simulink model "P2_SIL_Model_Diag"  (R2016a)
settings: Solver=ode2  StartTime=0.0  StopTime=Cycle_End  RelTol=1e-3
undefined symbols (not defined in the file): air, APP1_OOR, APP2_OOR, APP_Conversion_IN, APP_Mismatch, bms_inletair_temp, bms_maxchargecurrent, bms_maxdischargecurrent, BMS_Notfallkuehlung, BPP_Flt, cal, clt, ClutchEngag, CrankRequest, dcdc, eng, Engine, EngOverTemp, ENGTRQ_MSMCH_Degraded_CP, ENGTRQ_MSMCH_ErrCritical_CP, ENGTRQ_MSMCH_LimpHome_CP, EngTrqMismatch, env, ess, ESS, ESSOverTemp, fd, FFD, g, gb, Grade, IMG, KeyPos_Flt, KeyPosition, lib_APP_Conversion_IN, lib_ESS_plant_V1_2, lib_OBC_Manager, LossCAN, max_vehicle_rad_air_flow, MCUOverTemp, mot, MotDirMismatch, MotOverTemp, MotTrqMismatch, mph2kph, mph2ms, NeutralGear, obc, OBC_Manager, ParkGear, PRNDL_Flt, ReverseGear, RFD, rho, ShiftLeverPosition, sigbuilder_block, Speed, t_amb, time, tloop ... (+2)
libraries: simulink x104, EC2_libraries x12, Diagnostic x11, lib_CANerror_Detect x3, Utility x1
(part 3 of 11)

== system P2_SIL_Model_Diag/Actuators/CAN/HV_CAN/MCU ==
  In1 : Inport
  Bus Creator : BusCreator  Inputs=4
  Bus Selector : BusSelector  OutputSignals=MCU_CAN,Controls.Torque_Command,Controls.Inverter_Enable,Controls.ClutchEngage
  Out1 : Outport
  wires:
  In1/1 -> Bus Selector/1
  Bus Selector/1 -> Bus Creator/1  "<MCU_CAN>"
  Bus Selector/2 -> Bus Creator/2  "<Torque_Command>"
  Bus Creator/1 -> Out1/1
  Bus Selector/3 -> Bus Creator/3  "<Inverter_Enable>"
  Bus Selector/4 -> Bus Creator/4  "<ClutchEngage>"

== system P2_SIL_Model_Diag/Actuators/CAN/HV_CAN/OBC ==
  In1 : Inport
  Bus Selector : BusSelector  OutputSignals=OBC_CAN
  Out1 : Outport
  wires:
  In1/1 -> Bus Selector/1
  Bus Selector/1 -> Out1/1  "<OBC_CAN>"

== system P2_SIL_Model_Diag/Actuators/CAN/VEH_CAN/BCM ==
  In1 : Inport
  Bus Creator : BusCreator  Inputs=2
  Bus Selector : BusSelector  OutputSignals=Controls.powerMode,Controls.SysPwrMd
  Memory : Memory
  Out1 : Outport
  wires:
  In1/1 -> Bus Selector/1
  Bus Selector/1 -> Bus Creator/1  "<powerMode>"
  Bus Selector/2 -> Memory/1  "<SysPwrMd>"
  Bus Creator/1 -> Out1/1
  Memory/1 -> Bus Creator/2  "SysPwrMd"

== system P2_SIL_Model_Diag/Actuators/CAN/VEH_CAN/EBCM ==
  In1 : Inport
  Out1 : Outport
  wires:
  In1/1 -> Out1/1

== system P2_SIL_Model_Diag/Actuators/CAN/VEH_CAN/ICCM ==
  In1 : Inport
  Out1 : Outport
  wires:
  In1/1 -> Out1/1

== system P2_SIL_Model_Diag/Actuators/CAN/VEH_CAN/TCM ==
  In1 : Inport
  Bus Creator : BusCreator  Inputs=2
  Bus Selector : BusSelector  OutputSignals=Controls.VehSpdAvgDrvn_kph,Controls.AccPos_Perc
  Out1 : Outport
  wires:
  In1/1 -> Bus Selector/1
  Bus Selector/1 -> Bus Creator/1  "<VehSpdAvgDrvn_kph>"
  Bus Selector/2 -> Bus Creator/2  "<AccPos_Perc>"
  Bus Creator/1 -> Out1/1

== system P2_SIL_Model_Diag/Camaro Plant Model/Differential/Torque calculation/Blending (state dependent) ==
  Input : Inport
  Control (state) : Inport  Port=2
  Linear spline : Fcn  Expr=(u<xl)*yl + (xl<=u)*(u<xc)*((yc-yl)*(u-xl)/(xc-xl)+yl) + (xc<=u)*(u<xr)*((yc-yr)*(u-xr)/(xc-xr)+yr) + (xr<=u)*yr
  Product2 : Product  SaturateOnIntegerOverflow=on  InputSameDT=on  OutDataTypeStr=Inherit: Same as first input
  Output : Outport
  wires:
  Input/1 -> Product2/1
  Linear spline/1 -> Product2/2
  Product2/1 -> Output/1
  Control (state)/1 -> Linear spline/1

== system P2_SIL_Model_Diag/Camaro Plant Model/Differential/Torque calculation/Look-Up Table (2-D) ==
  Rows : Inport
  Cols : Inport  Port=2
  Look-Up Table (2-D) : Lookup2D  RowIndex=x  ColumnIndex=y  Table=t  SaturateOnIntegerOverflow=on  InputSameDT=on
  Out1 : Outport
  wires:
  Rows/1 -> Look-Up Table (2-D)/1
  Cols/1 -> Look-Up Table (2-D)/2
  Look-Up Table (2-D)/1 -> Out1/1

== system P2_SIL_Model_Diag/Camaro Plant Model/ESS/ESS/ESSThermal ==
  note: TempDeltaCdeg
  Resistance : Inport
  Current : Inport  Port=2
  BatteryMass : Constant  Value=ess.plant.init.bat_mass
  Constant : Constant  Value=0.01
  Divide : Product  Inputs=*/
  LowerLimit : Subsystem  mask{Lolimit=t_amb}
      mask prompts: Lolimit "Lower Limit:"
  LowerLimit1 : Subsystem  mask{Lolimit=70000}
      mask prompts: Lolimit "Lower Limit:"
  Memory : Memory  X0=t_amb
  Multiply : Product  Inputs=3
  Product : Product  RndMeth=Zero
  SpecificHeatCapBattery : Constant  Value=ess.plant.init.specific_heat
  Sum : Sum  Inputs=|++
  Sum1 : Sum  Inputs=-++  SaturateOnIntegerOverflow=on  InputSameDT=on  OutDataTypeStr=Inherit: Same as first input
  Sum2 : Sum  SaturateOnIntegerOverflow=on  InputSameDT=on  OutDataTypeStr=Inherit: Same as first input
  Switch4 : Switch  Threshold=1
  To Workspace3 : ToWorkspace  VariableName=ess_temp_hist  SampleTime=-1
      settings: Decimation=WORKSPACE_DECIMATION
  To_WHr1 : Gain  Gain=tloop  SaturateOnIntegerOverflow=on  OutDataTypeStr=Inherit: Same as input  ParamDataTypeStr=Inherit: Same as input
  To_WHr2 : Gain  Gain=5  SaturateOnIntegerOverflow=on  OutDataTypeStr=Inherit: Same as input  ParamDataTypeStr=Inherit: Same as input
  Temp[degC] : Outport
  wires:
  Sum2/1 -> Sum1/1
  Constant/1 -> Sum2/2  "NaturalCooling"
  [ESS_WEGPmp] -> Sum2/1
  To_WHr1/1 -> Divide/1  "d(Wh)"
  Current/1 -> Multiply/1, Multiply/2
  Resistance/1 -> Multiply/3
  Sum1/1 -> To_WHr1/1
  LowerLimit/1(Out) -> To Workspace3/1, Memory/1, Temp[degC]/1
  Memory/1 -> Sum/2
  Sum/1 -> LowerLimit/1(In)
  Divide/1 -> Sum/1
  BatteryMass/1 -> Product/1  "kg"
  SpecificHeatCapBattery/1 -> Product/2  "J/kg*K"
  Product/1 -> Divide/2
  Multiply/1 -> Sum1/2, To_WHr2/1  "J/s"
  Switch4/1 -> Sum1/3  "ResistiveFault"
  [ESSHighRes] -> Switch4/2, Switch4/3
  To_WHr2/1 -> LowerLimit1/1(In)
  LowerLimit1/1(Out) -> Switch4/1

== system P2_SIL_Model_Diag/Camaro Plant Model/ESS/ESS/LoadCharacteristics ==
  Current : Inport
  I*r : Product  RndMeth=Zero
  LowerLimit1 : Subsystem  mask{Lolimit=40}
      mask prompts: Lolimit "Lower Limit:"
  LowerLimit2 : Subsystem  mask{Lolimit=30}
      mask prompts: Lolimit "Lower Limit:"
  SOC Calculation : Subsystem
  Sum : Sum
  Switch1 : Switch  Threshold=1
  Switch2 : Switch
  Switch4 : Switch  Threshold=1
  To Workspace3 : ToWorkspace  VariableName=ess_voc_hist  SampleTime=-1
      settings: Decimation=WORKSPACE_DECIMATION
  To_WHr1 : Gain  Gain=10  SaturateOnIntegerOverflow=on  OutDataTypeStr=Inherit: Same as input  ParamDataTypeStr=Inherit: Same as input
  To_WHr2 : Gain  Gain=10  SaturateOnIntegerOverflow=on  OutDataTypeStr=Inherit: Same as input  ParamDataTypeStr=Inherit: Same as input
  To_WHr3 : Gain  Gain=1.01  SaturateOnIntegerOverflow=on  OutDataTypeStr=Inherit: Same as input  ParamDataTypeStr=Inherit: Same as input
  To_WHr4 : Gain  Gain=0.99  SaturateOnIntegerOverflow=on  OutDataTypeStr=Inherit: Same as input  ParamDataTypeStr=Inherit: Same as input
  resistor_charge (ohm) : Lookup  InputValues=ess.plant.init.bat_soc_idx  Table=ess.plant.init.bat_r_chg
  resistor_discharge (ohm) : Lookup  InputValues=ess.plant.init.bat_soc_idx  Table=ess.plant.init.bat_r_dis
  voc (volt) : Lookup  InputValues=ess.plant.init.bat_soc_idx  Table=ess.plant.init.bat_voc
  will use charge when >=0 : Switch
  Vterm : Outport
  Resistance : Outport  Port=2
  tag scope: SOC=global
  wires:
  To_WHr4/1 -> Switch2/1
  To_WHr3/1 -> Switch2/3
  Switch2/1 -> [Current_internal], SOC Calculation/1(Current)
  SOC Calculation/1(SOC) -> [SOC], voc (volt)/1, resistor_charge (ohm)/1, resistor_discharge (ohm)/1
  will use charge when >=0/1 -> Resistance/1, I*r/1
  I*r/1 -> Sum/2
  voc (volt)/1 -> [OCV], Sum/1, To Workspace3/1
  Sum/1 -> Vterm/1, [V_term]
  [ESSHighRes] -> Switch4/2, Switch1/2
  To_WHr2/1 -> LowerLimit1/1(In)
  resistor_charge (ohm)/1 -> Switch4/3, To_WHr2/1
  Switch4/1 -> will use charge when >=0/1  "ResistiveFault"
  Switch1/1 -> will use charge when >=0/3
  resistor_discharge (ohm)/1 -> Switch1/3, To_WHr1/1
  To_WHr1/1 -> LowerLimit2/1(In)
  LowerLimit1/1(Out) -> Switch4/1
  LowerLimit2/1(Out) -> Switch1/1
  Current/1 -> Switch2/2, To_WHr3/1, will use charge when >=0/2, I*r/2, [Current_term], To_WHr4/1

== system P2_SIL_Model_Diag/Camaro Plant Model/ESS/Inputs/CAN_fromHCU ==
  Bus Creator : BusCreator  Inputs=2
  Outputs : Outport
  wires:
  [HCU_to_HV_CAN] -> Bus Creator/1
  [HCU_to_EBCAN] -> Bus Creator/2
  Bus Creator/1 -> Outputs/1

== system P2_SIL_Model_Diag/Camaro Plant Model/ESS/Inputs/Digital_fromHCU ==
  Outputs : Outport
  wires:
  [Digital] -> Outputs/1

== system P2_SIL_Model_Diag/Camaro Plant Model/ESS/Soft BMS/BMS_06 ==
  Bus Creator8 : BusCreator  Inputs=9
  Constant2 : Constant  Value=0
  BMS_06 : Outport
  wires:
  Constant2/1 -> Bus Creator8/2  "BMS_SollVolumenStrom"
  Bus Creator8/1 -> BMS_06/1  "BMS_06"
  ? -> Bus Creator8/8
  ? -> Bus Creator8/6
  ? -> Bus Creator8/4
  ? -> Bus Creator8/3
  ? -> Bus Creator8/7
  ? -> Bus Creator8/9
  ? -> Bus Creator8/5

== system P2_SIL_Model_Diag/Camaro Plant Model/ESS/Soft BMS/BMS_07 ==
  Bus Creator8 : BusCreator  Inputs=9
  BMS_07 : Outport
  wires:
  ? -> Bus Creator8/5
  ? -> Bus Creator8/9
  ? -> Bus Creator8/7
  [BMS_Gesamtst_Spgfreiheit] -> Bus Creator8/1  "BMS_Gesamtst_Spgfreiheit"
  ? -> Bus Creator8/3
  ? -> Bus Creator8/4
  ? -> Bus Creator8/6
  ? -> Bus Creator8/8
  Bus Creator8/1 -> BMS_07/1  "BMS_07"
  ? -> Bus Creator8/2

== system P2_SIL_Model_Diag/Camaro Plant Model/ESS/Soft BMS/BMS_08  ==
  Bus Creator8 : BusCreator  Inputs=9
  BMS_08 : Outport
  wires:
  ? -> Bus Creator8/5
  ? -> Bus Creator8/9
  ? -> Bus Creator8/7
  [BMS_Temp_Zelle_Max] -> Bus Creator8/1  "BMS_Temp_Zelle_Max"
  ? -> Bus Creator8/3
  ? -> Bus Creator8/4
  ? -> Bus Creator8/6
  ? -> Bus Creator8/8
  Bus Creator8/1 -> BMS_08/1  "BMS_08"
  [BMS_Temp_Zelle_Min] -> Bus Creator8/2  "BMS_Temp_Zelle_Min"

== system P2_SIL_Model_Diag/Camaro Plant Model/ESS/Soft BMS/BMS_HYB_02 ==
  Bus Creator3 : BusCreator  Inputs=20
  Constant12 : Constant  Value=0
  Constant7 : Constant  Value=0
  Constant8 : Constant  Value=0
  Data Type Conversion4 : DataTypeConversion
  BMS_HYB_02 : Outport
  wires:
  Bus Creator3/1 -> BMS_HYB_02/1  "BMS_HYB_02"
  [BMS_IstModus] -> Bus Creator3/1  "BMS_IstModus"
  [BMS_Gesamtst_Spgfreiheit] -> Bus Creator3/3  "BMS_Status_Spannungsfreiheit"
  [BMS_Fehler_Notabschaltung_Crash] -> Bus Creator3/6  "BMS_Fehler_HVBattAbschaltung"
  Constant7/1 -> Bus Creator3/7  "BMS_Fehler_HVBattAbschaltung_Anf"
  [BMS_Notfallkuehlung] -> Bus Creator3/2  "BMS_Notfallkuehlung"
  Constant8/1 -> Bus Creator3/8  "BMS_Fehler_Isolation"
  [BMS_Fehler_Notabschaltung_Crash] -> Bus Creator3/5  "BMS_Fehler_Notabschaltung_Crash"
  [BMS_Gesamtst_Spgfreiheit] -> Bus Creator3/4  "BMS_Status_Spgfreiheit"
  [BMS_Fehler_Pilot] -> Bus Creator3/9  "BMS_Fehler_Pilot"
  [BMS_IstStrom] -> Bus Creator3/10  "BMS_IstStrom"
  [BMS_Fehler_HS_offen] -> Bus Creator3/11  "BMS_Fehler_HS_offen"
  [BMS_Fehler_verschweisst] -> Bus Creator3/12  "BMS_Fehler_HS_verschweisst"
  [BMS_IstSpannung] -> Bus Creator3/13  "BMS_IstSpannung"
  Constant12/1 -> Bus Creator3/14  "BMS_Fehler_Kaltstartleistung"
  [BMS_Init_abgeschlossen] -> Bus Creator3/15  "BMS_Init_abgescholssen"
  [BMS_Fehler_Notabschaltung_Pilot] -> Bus Creator3/16  "BMS_Fehler_Notabschaltung_Pilot"
  [BMS_SleepInd] -> Bus Creator3/17  "BMS_SleepInd"
  [MO_BMS_Sollmodus] -> Data Type Conversion4/1  "MO_BMS_Sollmodus"
  Data Type Conversion4/1 -> Bus Creator3/18  "MO_BMS_Sollmodus"

== system P2_SIL_Model_Diag/Camaro Plant Model/ESS/Soft BMS/BMS_HYB_03 ==
  Bus Creator3 : BusCreator  Inputs=10
  BMS_HYB_03 : Outport
  wires:
  [BMS_SOC] -> Bus Creator3/1  "BMS_SOC"
  Bus Creator3/1 -> BMS_HYB_03/1  "BMS_HYB_03"

== system P2_SIL_Model_Diag/Camaro Plant Model/ESS/Soft BMS/BMS_HYB_04 ==
  Bus Creator6 : BusCreator  Inputs=9
  Constant : Constant
  Constant1 : Constant  Commented=on  Value=bms_maxdischargecurrent
  Constant2 : Constant
  Constant3 : Constant  Commented=on  Value=bms_maxchargecurrent
  BMS_HYB_04 : Outport
  wires:
  Constant/1 -> Bus Creator6/1  "BMS_MaxDyn_LadeStrom"
  Bus Creator6/1 -> BMS_HYB_04/1  "BMS_HYB_04"
  ? -> Bus Creator6/6
  ? -> Bus Creator6/4
  ? -> Bus Creator6/5
  ? -> Bus Creator6/8
  ? -> Bus Creator6/9
  ? -> Bus Creator6/7
  [BMS_Spannung_ZwKr] -> Bus Creator6/3  "BMS_Spannung_ZwKr"
  Constant2/1 -> Bus Creator6/2

== system P2_SIL_Model_Diag/Camaro Plant Model/ESS/Soft BMS/BMS_HYB_06 ==
  Bus Creator6 : BusCreator  Inputs=9
  Constant1 : Constant  Value=430
  Constant2 : Constant  Value=291
  Constant3 : Constant  Value=0
  Constant4 : Constant  Commented=on  Value=bms_inletair_temp
  Constant5 : Constant  Value=20
  BMS_HYB_06 : Outport
  wires:
  Constant1/1 -> Bus Creator6/2  "BMS_Max_LadeSpannung"
  ? -> Bus Creator6/7
  ? -> Bus Creator6/9
  ? -> Bus Creator6/8
  Constant2/1 -> Bus Creator6/3  "BMS_Min_EntladeSpannung"
  ? -> Bus Creator6/6
  Bus Creator6/1 -> BMS_HYB_06/1  "BMS_HYB_06"
  Constant3/1 -> Bus Creator6/1  "BMS_Balancing_Anf"
  [BMS_Temperatur] -> Bus Creator6/4  "BMS_Temperatur"
  Constant5/1 -> Bus Creator6/5  "BMS_Temperatur_Ansaugluft"

== system P2_SIL_Model_Diag/Camaro Plant Model/ESS/Soft BMS/BMS_HYB_07 ==
  Bus Creator6 : BusCreator  Inputs=9
  BMS_HYB_07 : Outport
  wires:
  [BMS_Temperierung_Anf] -> Bus Creator6/1  "BMS_Temperierung_Anf"
  Bus Creator6/1 -> BMS_HYB_07/1  "BMS_HYB_07"
  ? -> Bus Creator6/6
  ? -> Bus Creator6/4
  ? -> Bus Creator6/5
  ? -> Bus Creator6/8
  ? -> Bus Creator6/9
  ? -> Bus Creator6/7

== system P2_SIL_Model_Diag/Camaro Plant Model/ESS/Soft BMS/BMS_Hybrid_01 ==
  Bus Creator8 : BusCreator  Inputs=1
  BMS_Hybrid_01 : Outport
  wires:
  Bus Creator8/1 -> BMS_Hybrid_01/1  "BMS_Hybrid_01"
  [BMS_HYB_Kuehlung_Anf] -> Bus Creator8/1  "BMS_HYB_Kuehlung_Anf"

== system P2_SIL_Model_Diag/Camaro Plant Model/ESS/Soft BMS/Energy Consumption ==
  Current : Inport
  Voltage : Inport  Port=2
  Divide : Product  Inputs=*/
  Divide by zero : Subsystem
  Gain : Gain  Gain=mph2kph
  Initial Current1 : Memory  InheritSampleTime=on
  Multiply : Product  Inputs=**
  Sum5 : Sum  Inputs=|++  SaturateOnIntegerOverflow=on  InputSameDT=on  OutDataTypeStr=Inherit: Same as first input
  To Workspace4 : ToWorkspace  VariableName=ess_wh_per_km  SampleTime=-1
      settings: Decimation=WORKSPACE_DECIMATION
  To_WHr1 : Gain  Gain=tloop/3600  SaturateOnIntegerOverflow=on  OutDataTypeStr=Inherit: Same as input  ParamDataTypeStr=Inherit: Same as input
  wires:
  Current/1 -> Multiply/1
  Voltage/1 -> Multiply/2
  Multiply/1 -> To_WHr1/1  "Power"
  To_WHr1/1 -> Sum5/1  "d(Wh)"
  Sum5/1 -> Initial Current1/1  "Wh"
  Initial Current1/1 -> Sum5/2, Divide/1  "Wh"
  [veh_dist_miles] -> Gain/1  "mi"
  Divide/1 -> To Workspace4/1  "Wh/km"
  Gain/1 -> Divide by zero/1(In1)  "km"
  Divide by zero/1(Out1) -> Divide/2

== system P2_SIL_Model_Diag/Camaro Plant Model/ESS/Soft BMS/HV_Netz status ==
  ess_vbat : Inport
  Constant3 : Constant  Value=2
  Constant4 : Constant
  Constant5 : Constant  Value=0
  Constant6 : Constant  Value=0
  Memory : Memory
  Memory1 : Memory
  Switch : Switch  Criteria=u2 > Threshold  Threshold=20
  Switch1 : Switch  Threshold=1
  Switch2 : Switch  Threshold=7
  BMS_Spannung_Zwkr : Outport
  BMS_Gesamtst_Spgfreiheit : Outport  Port=2
  wires:
  Constant5/1 -> Switch1/3
  [BMS_IstModus] -> Switch1/2, Switch2/2
  Switch1/1 -> Memory/1
  Constant6/1 -> Switch2/1
  Switch2/1 -> Memory1/1
  Constant4/1 -> Switch/3
  Switch/1 -> BMS_Gesamtst_Spgfreiheit/1
  Constant3/1 -> Switch/1
  ess_vbat/1 -> Switch1/1
  Memory/1 -> Switch2/3
  Memory1/1 -> BMS_Spannung_Zwkr/1, Switch/2

== system P2_SIL_Model_Diag/Camaro Plant Model/ESS/Soft BMS/Limits ==
  vcell : Inport
  Average Current : Subsystem
  Compare To Constant1 : simulink/Logic and Bit Operations/Compare To Constant  relop=<=  const=3.0  OutDataTypeStr=boolean
  Compare To Constant2 : simulink/Logic and Bit Operations/Compare To Constant  relop=<=  const=3.0  OutDataTypeStr=boolean
  Constant3 : Constant  Value=25
  Derate : Subsystem
  Derate2 : Subsystem
  Gain : Gain  Gain=1/1.9
  Gain1 : Gain  Gain=1/1.9
  To Workspace10 : ToWorkspace  VariableName=ess_dis_max_current_underated  SampleTime=-1
      settings: Decimation=WORKSPACE_DECIMATION
  To Workspace3 : ToWorkspace  VariableName=ess_dis_max  SampleTime=-1
      settings: Decimation=WORKSPACE_DECIMATION
  To Workspace4 : ToWorkspace  VariableName=ess_chg_max  SampleTime=-1
      settings: Decimation=WORKSPACE_DECIMATION
  To Workspace9 : ToWorkspace  VariableName=ess_chg_max_current_underated  SampleTime=-1
      settings: Decimation=WORKSPACE_DECIMATION
  bcm_chg_max_tbl : Lookup2D  RowIndex=ess.plant.init.limit.idx1_soc  ColumnIndex=ess.plant.init.limit.idx2_temp  Table=ess.plant.init.max_charge_limit
  bcm_dis_max_tbl : Lookup2D  RowIndex=ess.plant.init.limit.idx1_soc  ColumnIndex=ess.plant.init.limit.idx2_temp  Table=ess.plant.init.max_discharge_limit
  bcm_dis_max : Outport
  bcm_chg_max : Outport  Port=2
  Discharge Buffer : Outport  Port=3
  Charge Buffer : Outport  Port=4
  t_coolant : Outport  Port=5
  undervolt : Outport  Port=6
  overvolt : Outport  Port=7
  tag scope: bcm_chg_max=global
  wires:
  [BMS_Temperatur] -> bcm_chg_max_tbl/2, bcm_dis_max_tbl/2, Average Current/2(Temp)
  bcm_dis_max_tbl/1 -> Gain/1
  Derate/1(Derate) -> bcm_dis_max/1, To Workspace3/1
  bcm_chg_max_tbl/1 -> Gain1/1  "bcm_chg_max"
  Derate2/1(Derate) -> To Workspace4/1, [bcm_chg_max], bcm_chg_max/1
  [BMS_SOC] -> Average Current/1(SOC), bcm_dis_max_tbl/1, bcm_chg_max_tbl/1
  Average Current/1(Discharge Buffer) -> Derate/2(Buffer), Discharge Buffer/1
  Average Current/2(Discharge Cont) -> Derate/3(Cont Current)
  Average Current/3(Charge Buffer) -> Derate2/1(Buffer), Charge Buffer/1
  Average Current/4(Charge Cont) -> Derate2/2(Cont Current)
  vcell/1 -> Compare To Constant1/1, Compare To Constant2/1
  Constant3/1 -> t_coolant/1
  Compare To Constant2/1 -> overvolt/1
  Compare To Constant1/1 -> undervolt/1
  Gain/1 -> Derate/1(Current Limit), To Workspace10/1
  Gain1/1 -> To Workspace9/1, Derate2/3(Current Limit)

== system P2_SIL_Model_Diag/Camaro Plant Model/ESS/Soft BMS/NMH_BMS ==
  Bus Creator8 : BusCreator  Inputs=9
  NMH_BMS : Outport
  wires:
  [NMH_BMS_Car_WakeUp] -> Bus Creator8/5  "NMH_BMS_Car_WakeUp"
  ? -> Bus Creator8/9
  ? -> Bus Creator8/7
  [NMH_BMS_Normal_Mode_1] -> Bus Creator8/1  "NMH_BMS_Normal_Mode_1"
  [NMH_BMS_Start_2] -> Bus Creator8/4  "NMH_BMS_Start_2"
  ? -> Bus Creator8/6
  ? -> Bus Creator8/8
  Bus Creator8/1 -> NMH_BMS/1  "NMH_BMS"
  [NMH_BMS_Normal_Mode_2] -> Bus Creator8/2  "NMH_BMS_Normal_Mode_2"
  [NMH_BMS_Start_1] -> Bus Creator8/3  "NMH_BMS_Start_1"

== system P2_SIL_Model_Diag/Camaro Plant Model/ESS/Soft BMS/NoiseAdd ==
  In : Inport
  Random Number : RandomNumber  Variance=0.1  SampleTime=tloop
  Rate Transition : RateTransition
  Sum : Sum  Inputs=|++
  Out : Outport
  wires:
  Random Number/1 -> Rate Transition/1
  In/1 -> Sum/1
  Sum/1 -> Out/1
  Rate Transition/1 -> Sum/2

== system P2_SIL_Model_Diag/Camaro Plant Model/ESS/Soft BMS/RollingAliveCnt ==
  Constant : Constant
  Rolling Alive Counter : Stateflow chart  TreatAsAtomicUnit=on
  Switch : Switch  Criteria=u2 > Threshold
  Out1 : Outport
  wires:
  Switch/1 -> Out1/1
  [BMS_CAN_fault] -> Switch/2
  Rolling Alive Counter/1(RollingAliveCnt) -> Switch/3
  Constant/1 -> Switch/1

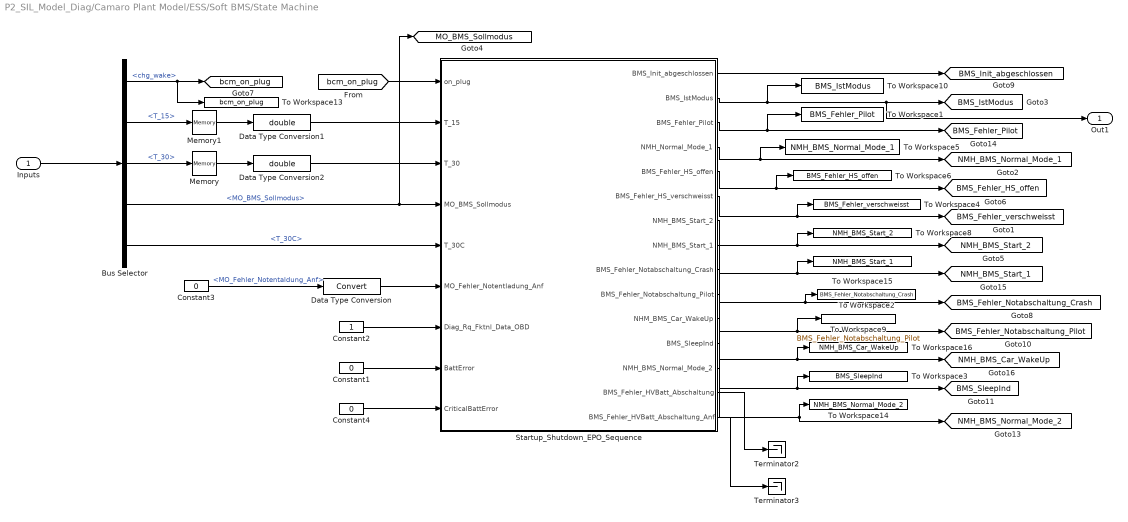
== system P2_SIL_Model_Diag/Camaro Plant Model/ESS/Soft BMS/State Machine ==
  Inputs : Inport
  Bus Selector : BusSelector  OutputSignals=Digital.chg_wake,Digital.T_15,Digital.T_30,CAN.to HV_CAN.to_BMS_Hybrid.MO_BMS_Sollmodus,Digital.T_30C
  Constant1 : Constant  Value=0  OutDataTypeStr=boolean
  Constant2 : Constant  OutDataTypeStr=boolean
  Constant3 : Constant  Value=0  OutDataTypeStr=boolean
  Constant4 : Constant  Value=0  OutDataTypeStr=boolean
  Data Type Conversion : DataTypeConversion
  Data Type Conversion1 : DataTypeConversion  OutDataTypeStr=double
  Data Type Conversion2 : DataTypeConversion  OutDataTypeStr=double
  Memory : Memory
  Memory1 : Memory
  Startup_Shutdown_EPO_Sequence : Stateflow chart  TreatAsAtomicUnit=on
  Terminator2 : Terminator
  Terminator3 : Terminator
  To Workspace1 : ToWorkspace  VariableName=BMS_Fehler_Pilot  SampleTime=-1
      settings: Decimation=WORKSPACE_DECIMATION
  To Workspace10 : ToWorkspace  VariableName=BMS_IstModus  SampleTime=-1
      settings: Decimation=WORKSPACE_DECIMATION
  To Workspace13 : ToWorkspace  VariableName=bcm_on_plug  SampleTime=-1
      settings: Decimation=WORKSPACE_DECIMATION
  To Workspace14 : ToWorkspace  VariableName=NMH_BMS_Normal_Mode_2  SampleTime=-1
      settings: Decimation=WORKSPACE_DECIMATION
  To Workspace15 : ToWorkspace  VariableName=NMH_BMS_Start_1  SampleTime=-1
      settings: Decimation=WORKSPACE_DECIMATION
  To Workspace16 : ToWorkspace  VariableName=NMH_BMS_Car_WakeUp  SampleTime=-1
      settings: Decimation=WORKSPACE_DECIMATION
  To Workspace2 : ToWorkspace  VariableName=BMS_Fehler_Notabschaltung_Crash  SampleTime=-1
      settings: Decimation=WORKSPACE_DECIMATION
  To Workspace3 : ToWorkspace  VariableName=BMS_SleepInd  SampleTime=-1
      settings: Decimation=WORKSPACE_DECIMATION
  To Workspace4 : ToWorkspace  VariableName=BMS_Fehler_verschweisst  SampleTime=-1
      settings: Decimation=WORKSPACE_DECIMATION
  To Workspace5 : ToWorkspace  VariableName=NMH_BMS_Normal_Mode_1  SampleTime=-1
      settings: Decimation=WORKSPACE_DECIMATION
  To Workspace6 : ToWorkspace  VariableName=BMS_Fehler_HS_offen  SampleTime=-1
      settings: Decimation=WORKSPACE_DECIMATION
  To Workspace8 : ToWorkspace  VariableName=NMH_BMS_Start_2  SampleTime=-1
      settings: Decimation=WORKSPACE_DECIMATION
  To Workspace9 : ToWorkspace  VariableName=BMS_Fehler_Notabschaltung_Pilot  SampleTime=-1
      settings: Decimation=WORKSPACE_DECIMATION
  Out1 : Outport
  tag scope: BMS_Fehler_HS_offen=global, BMS_Fehler_Notabschaltung_Crash=global, BMS_Fehler_Notabschaltung_Pilot=global, BMS_Fehler_Pilot=global, BMS_Fehler_verschweisst=global, BMS_Init_abgeschlossen=global, BMS_IstModus=global, BMS_SleepInd=global, MO_BMS_Sollmodus=global, NMH_BMS_Car_WakeUp=global, NMH_BMS_Normal_Mode_1=global, NMH_BMS_Normal_Mode_2=global, NMH_BMS_Start_1=global, NMH_BMS_Start_2=global, bcm_on_plug=global
  wires:
  Bus Selector/3 -> Memory/1  "<T_30>"
  Bus Selector/1 -> To Workspace13/1, [bcm_on_plug]  "<chg_wake>"
  Startup_Shutdown_EPO_Sequence/12(BMS_SleepInd) -> To Workspace3/1, [BMS_SleepInd]
  Startup_Shutdown_EPO_Sequence/5(BMS_Fehler_HS_offen) -> To Workspace6/1, [BMS_Fehler_HS_offen]
  Startup_Shutdown_EPO_Sequence/10(BMS_Fehler_Notabschaltung_Pilot) -> To Workspace9/1, [BMS_Fehler_Notabschaltung_Pilot]
  Startup_Shutdown_EPO_Sequence/9(BMS_Fehler_Notabschaltung_Crash) -> To Workspace2/1, [BMS_Fehler_Notabschaltung_Crash]
  Startup_Shutdown_EPO_Sequence/4(NMH_Normal_Mode_1) -> To Workspace5/1, [NMH_BMS_Normal_Mode_1]
  Startup_Shutdown_EPO_Sequence/6(BMS_Fehler_HS_verschweisst) -> [BMS_Fehler_verschweisst], To Workspace4/1
  Bus Selector/2 -> Memory1/1  "<T_15>"
  Startup_Shutdown_EPO_Sequence/2(BMS_IstModus) -> Out1/1, [BMS_IstModus], To Workspace10/1
  Startup_Shutdown_EPO_Sequence/1(BMS_Init_abgeschlossen) -> [BMS_Init_abgeschlossen]
  Startup_Shutdown_EPO_Sequence/3(BMS_Fehler_Pilot) -> To Workspace1/1, [BMS_Fehler_Pilot]
  Startup_Shutdown_EPO_Sequence/13(NMH_BMS_Normal_Mode_2) -> To Workspace14/1, [NMH_BMS_Normal_Mode_2]
  Startup_Shutdown_EPO_Sequence/7(NMH_BMS_Start_2) -> To Workspace8/1, [NMH_BMS_Start_2]
  Startup_Shutdown_EPO_Sequence/8(NMH_BMS_Start_1) -> [NMH_BMS_Start_1], To Workspace15/1
  Startup_Shutdown_EPO_Sequence/11(NHM_BMS_Car_WakeUp) -> To Workspace16/1, [NMH_BMS_Car_WakeUp]
  [bcm_on_plug] -> Startup_Shutdown_EPO_Sequence/1(on_plug)
  Bus Selector/5 -> Startup_Shutdown_EPO_Sequence/5(T_30C)  "<T_30C>"
  Constant3/1 -> Data Type Conversion/1  "<MO_Fehler_Notentaldung_Anf>"
  Constant1/1 -> Startup_Shutdown_EPO_Sequence/8(BattError)
  Constant2/1 -> Startup_Shutdown_EPO_Sequence/7(Diag_Rq_Fktnl_Data_OBD)
  Constant4/1 -> Startup_Shutdown_EPO_Sequence/9(CriticalBattError)
  Startup_Shutdown_EPO_Sequence/14(BMS_Fehler_HVBatt_Abschaltung) -> Terminator2/1
  Startup_Shutdown_EPO_Sequence/15(BMS_Fehler_HVBatt_Abschaltung_Anf) -> Terminator3/1
  Inputs/1 -> Bus Selector/1
  Data Type Conversion/1 -> Startup_Shutdown_EPO_Sequence/6(MO_Fehler_Notentladung_Anf)
  Data Type Conversion1/1 -> Startup_Shutdown_EPO_Sequence/2(T_15)
  Data Type Conversion2/1 -> Startup_Shutdown_EPO_Sequence/3(T_30)
  Memory/1 -> Data Type Conversion2/1
  Memory1/1 -> Data Type Conversion1/1
  Bus Selector/4 -> [MO_BMS_Sollmodus], Startup_Shutdown_EPO_Sequence/4(MO_BMS_Sollmodus)  "<MO_BMS_Sollmodus>"

== system P2_SIL_Model_Diag/Camaro Plant Model/ESS/Soft BMS/Temperature Management ==
  ess_temp : Inport
  Constant : Constant
  Constant1 : Constant  Value=3
  Constant2 : Constant  Commented=on  Value=BMS_Notfallkuehlung
  Constant3 : Constant
  Switch : Switch
  tag scope: BMS_HYB_Kuehlung_Anf=global, BMS_Temperatur=global, BMS_Temperierung_Anf=global
  wires:
  Constant/1 -> Switch/1
  ess_temp/1 -> [BMS_Temperatur], Switch/2
  Switch/1 -> [BMS_HYB_Kuehlung_Anf], [BMS_Temperierung_Anf]
  Constant1/1 -> Switch/3
  Constant3/1 -> [BMS_Notfallkuehlung]

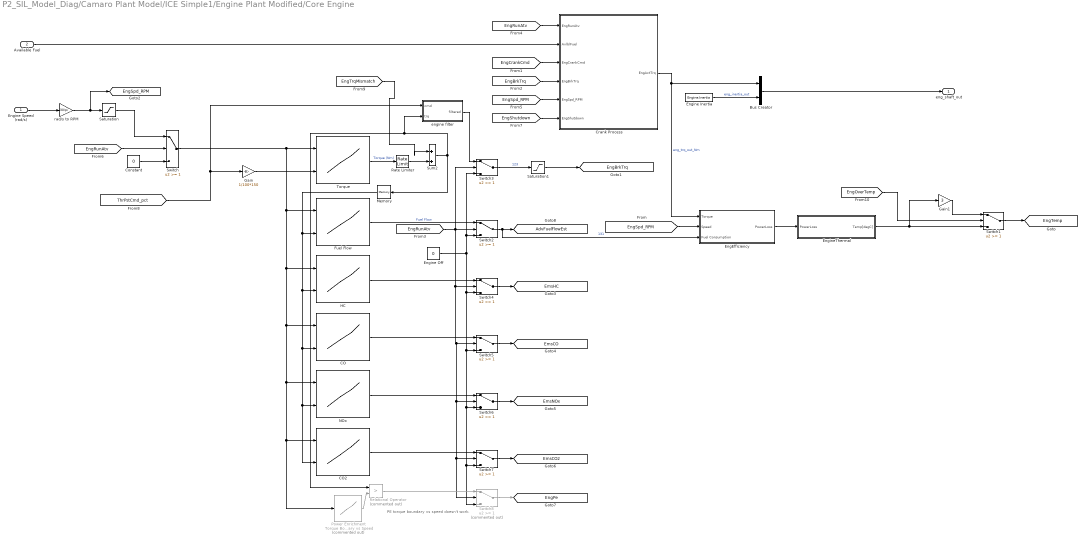
== system P2_SIL_Model_Diag/Camaro Plant Model/ICE Simple1/Engine Plant Modified/Core Engine ==
  note: PE torque boundary vs speed doesn't work.
  Engine Speed (rad/s) : Inport
  Available Fuel : Inport  Port=2
  Bus Creator : BusCreator  Inputs=2
  CO : Lookup2D  RowIndex=Engine.Engine.Emissions.SPEED  ColumnIndex=Engine.Engine.Emissions.TQ  Table=Engine.Engine.Emissions.CO/1000  LookUpMeth=Interpolation-Use End Values
  CO2 : Lookup2D  RowIndex=Engine.Engine.Emissions.SPEED  ColumnIndex=Engine.Engine.Emissions.TQ  Table=Engine.Engine.Emissions.CO2/1000  LookUpMeth=Interpolation-Use End Values
  Constant : Constant  Value=0
  Crank Process : Stateflow chart  TreatAsAtomicUnit=on
  EngEfficiency : Subsystem
  Engine Inertia : Constant  Value=Engine.Inertia
  "Engine Off  " : Constant  Value=0
  EngineThermal : Subsystem
  Fuel Flow : Lookup2D  RowIndex=Engine.Engine.FuelFlow.SPEED  ColumnIndex=Engine.Engine.FuelFlow.TQ  Table=Engine.Engine.FuelFlow.FuelFlow  LookUpMeth=Interpolation-Use End Values
  Gain : Gain  Gain=1/100*150
  Gain1 : Gain  Gain=3
  HC : Lookup2D  RowIndex=Engine.Engine.Emissions.SPEED  ColumnIndex=Engine.Engine.Emissions.TQ  Table=Engine.Engine.Emissions.HC/1000  LookUpMeth=Interpolation-Use End Values
  Memory : Memory
  NOx : Lookup2D  RowIndex=Engine.Engine.Emissions.SPEED  ColumnIndex=Engine.Engine.Emissions.TQ  Table=Engine.Engine.Emissions.NOx/1000  LookUpMeth=Interpolation-Use End Values
  Power Enrichment Torque Boundary vs Speed : Lookup_n-D  Commented=on  NumberOfTableDimensions=1  BreakpointsForDimension1=Engine.Engine.PEBound.SPEED  Table=Engine.Engine.PEBound.PEBound  ExtrapMethod=Clip  InternalRulePriority=Speed  RndMeth=Simplest  InputSameDT=on
  Rate Limiter : RateLimiter  RisingSlewLimit=230  FallingSlewLimit=-230  SampleTimeMode=inherited
  Relational Operator : RelationalOperator  Commented=on  Operator=>  OutDataTypeStr=boolean
  Saturation : Saturate  UpperLimit=max(Engine.Engine.TQ.SPEED)  LowerLimit=0
  Saturation1 : Saturate  UpperLimit=Engine.Max_Torque  LowerLimit=0
  Sum2 : Sum  Inputs=|++
  Switch{,1..7} (8 alike) : Switch  Threshold=1
  Switch8 : Switch  Commented=on  Threshold=1
  Torque : Lookup2D  RowIndex=Engine.Engine.TQ.SPEED  ColumnIndex=Engine.Engine.TQ.MAF  Table=Engine.Engine.TQ.TQ  LookUpMeth=Interpolation-Use End Values
  engine filter : Subsystem
  rad/s to RPM : Gain  Gain=30/pi
  eng_shaft_out : Outport
  tag scope: AdvFuelFlowEst=global, EmsCO2=global, EmsCO=global, EmsHC=global, EmsNOx=global, EngBrkTrq=global, EngPe=global, EngSpd_RPM=global, EngTemp=global
  wires:
  [ThrPstCmd_pct] -> engine filter/1(cmd), Gain/1
  Gain/1 -> Torque/2
  [EngShutdown] -> Crank Process/6(EngShutdown)
  Saturation/1 -> Switch/1
  [EngSpd_RPM] -> Crank Process/5(EngSpd_RPM)
  [EngCrankCmd] -> Crank Process/3(EngCrankCmd)
  [EngBrkTrq] -> Crank Process/4(EngBrkTrq)
  [EngRunAtv] -> Crank Process/1(EngRunAtv)
  Switch8/1 -> [EngPe]
  Switch7/1 -> [EmsCO2]
  CO2/1 -> Switch7/1
  Switch6/1 -> [EmsNOx]
  NOx/1 -> Switch6/1
  Switch5/1 -> [EmsCO]
  "Engine Off  "/1 -> Switch5/3, Switch7/3, Switch8/3, Switch6/3, Switch4/3, Switch2/3, Switch3/3
  [EngRunAtv] -> Switch5/2, Switch6/2, Switch7/2, Switch8/2, Switch4/2, Switch2/2, Switch3/2
  CO/1 -> Switch5/1
  Relational Operator/1 -> Switch8/1
  Switch4/1 -> [EmsHC]
  Switch3/1 -> Saturation1/1  "123"
  Available Fuel/1 -> Crank Process/2(AvlblFuel)
  Switch2/1 -> EngEfficiency/3(Fuel Consumption), [AdvFuelFlowEst]  "131"
  Fuel Flow/1 -> Switch2/1  "Fuel Flow"
  Power Enrichment Torque Boundary vs Speed/1 -> Relational Operator/2
  HC/1 -> Switch4/1
  Crank Process/1(EngActTrq) -> Bus Creator/1, EngEfficiency/1(Torque)  "eng_trq_out_Nm"
  Engine Inertia/1 -> Bus Creator/2  "eng_inertia_out"
  Bus Creator/1 -> eng_shaft_out/1
  [EngRunAtv] -> Switch/2
  Constant/1 -> Switch/3
  rad/s to RPM/1 -> [EngSpd_RPM], Saturation/1
  EngEfficiency/1(PowerLoss) -> EngineThermal/1(PowerLoss)
  Memory/1 -> CO2/2, NOx/2, CO/2, HC/2, Fuel Flow/2
  EngineThermal/1(Temp[degC]) -> Gain1/1, Switch1/3
  Engine Speed (rad/s)/1 -> rad/s to RPM/1
  Switch/1 -> Torque/1, Fuel Flow/1, HC/1, CO/1, NOx/1, CO2/1, Power Enrichment Torque Boundary vs Speed/1
  Sum2/1 -> Memory/1, Relational Operator/1, engine filter/2(trq)
  [EngSpd_RPM] -> EngEfficiency/2(Speed)
  Saturation1/1 -> [EngBrkTrq]
  [EngTrqMismatch] -> Sum2/1
  [EngOverTemp] -> Switch1/2
  Gain1/1 -> Switch1/1
  Switch1/1 -> [EngTemp]
  engine filter/1(filtered) -> Switch3/1
  Torque/1 -> Rate Limiter/1  "Torque (Nm)"
  Rate Limiter/1 -> Sum2/2

== system P2_SIL_Model_Diag/Camaro Plant Model/ICE Simple1/Engine Plant Modified/ECU Actuators ==
  In1 : Inport
  Bus Selector : BusSelector  OutputSignals=ThrPosCmd_%,Eng12vStrtrMtrCmmdOn,EngRunAtv,FuelPumpEnable,EngShutdown,Eng_Temp,fan_cmd,VehSpdAvgDrvn
  Out1 : Outport
  Out2 : Outport  Port=2
  Out3 : Outport  Port=3
  Out4 : Outport  Port=4
  Out5 : Outport  Port=5
  Out6 : Outport  Port=6
  Out7 : Outport  Port=7
  Out8 : Outport  Port=8
  wires:
  Bus Selector/5 -> Out5/1  "<EngShutdown>"
  Bus Selector/4 -> Out4/1  "<FuelPumpEnable>"
  In1/1 -> Bus Selector/1
  Bus Selector/1 -> Out1/1  "<ThrPosCmd_%>"
  Bus Selector/2 -> Out2/1  "<Eng12vStrtrMtrCmmdOn>"
  Bus Selector/3 -> Out3/1  "<EngRunAtv>"
  Bus Selector/6 -> Out6/1  "<Eng_Temp>"
  Bus Selector/7 -> Out7/1  "<fan_cmd>"
  Bus Selector/8 -> Out8/1  "<VehSpdAvgDrvn>"

== system P2_SIL_Model_Diag/Camaro Plant Model/ICE Simple1/Engine Plant Modified/ECU Sensors ==
  In1 : Inport
  In2 : Inport  Port=2
  In3 : Inport  Port=3
  In4 : Inport  Port=4
  In5 : Inport  Port=5
  In6 : Inport  Port=6
  In7 : Inport  Port=7
  In8 : Inport  Port=8
  In9 : Inport  Port=9
  In10 : Inport  Port=10
  Bus Creator : BusCreator  Inputs=10
  Memory : Memory
  Out1 : Outport
  wires:
  In9/1 -> Bus Creator/9  "NOx_g/s"
  In1/1 -> Bus Creator/1  "EngActStdyStTorq_Nm"
  In2/1 -> Bus Creator/2  "EngSpd_RPM"
  In3/1 -> Bus Creator/3  "EngFuelFlow_g/s"
  In4/1 -> Bus Creator/4  "FuelLevelPct"
  In5/1 -> Bus Creator/5  "PE_0_1"
  In6/1 -> Bus Creator/6  "HC_g/s"
  In7/1 -> Bus Creator/7  "CO_g/s"
  Bus Creator/1 -> Memory/1
  In8/1 -> Bus Creator/8  "CO2_g/s"
  In10/1 -> Bus Creator/10  "Eng_Temp"
  Memory/1 -> Out1/1

== system P2_SIL_Model_Diag/Camaro Plant Model/ICE Simple1/Engine Plant Modified/Fuel Supply ==
  0 to 100 : Saturate
  Fuel Pump Disable : Constant  Value=0
  Fuel Volumn : Constant  Value=Engine.Fuel.Initial_Volumn
  Integrator : Integrator  LimitOutput=on  UpperSaturationLimit=Engine.FuelTank.Volume  LowerSaturationLimit=0
  L to % : Gain  Gain=100/Engine.FuelTank.Volume
  Sum : Sum  Inputs=+-
  Switch : Switch  Threshold=1
  g to L : Gain  Gain=1/Engine.Fuel.Density/1000
  Available Fuel : Outport
  tag scope: FuelLevelPct=global
  wires:
  0 to 100/1 -> [FuelLevelPct]
  L to %/1 -> 0 to 100/1
  Fuel Pump Disable/1 -> Switch/3
  g to L/1 -> Switch/1
  Integrator/1 -> g to L/1
  [AdvFuelFlowEst] -> Integrator/1
  [FuelPumpEnable] -> Switch/2
  Sum/1 -> Available Fuel/1, L to %/1
  Switch/1 -> Sum/2
  Fuel Volumn/1 -> Sum/1

== system P2_SIL_Model_Diag/Camaro Plant Model/ICE Simple1/Engine Plant Modified/Radiator ==
  note: Calculation of max air flow:
      |
      | The air flow reach the max in the scenario that only fan rejects all the heat coolant brings in
      |
      | The regular max CFM of a vehicle radiator fan is about 2000
      |
      | CFM=1.76* Q/delta T_air
      |
      | Where Q is the max amount of heat from coolant, assume that the max temperature drop of coolant
      | through radiator is 10 deg C
      |
      | Q= Mc_coolant* Cp_coolant* delta T_coolant=3500*0.26*10=9100w
      |
      | delta T_air=1.76*Q/CFM=1.76*9100/2000=8 degC
      |
      | Max Mc_air=Q/(Cp_air*delta T_air)=9100/(1006*8)=1.13 kg/s
  EngCltTmp : Inport
  Fans : Inport  Port=2
  " " : Product  Inputs=**
  " " : Gain  Gain=0.05
  Ambient Temp : Constant  Value=env.init.T_ambiant
  Compare To Zero : simulink/Logic and Bit Operations/Compare To Zero  relop===  OutDataTypeStr=uint8
  Constant : Constant
  Cp of Air : Constant  Value=air.init.specific_heat
  Cp of Air1 : Constant  Value=air.init.specific_heat
  Data Type Conversion1 : DataTypeConversion
  Divide by Zero Fix : Subsystem
  "Eng Mc=Q/(Cp*delta T) " : Product  Inputs=*/
  Q=Mc_air*Cp_air*delta T : Product  Inputs=***
  Saturation : Saturate  UpperLimit=max_vehicle_rad_air_flow  LowerLimit=-1
  Sum3 : Sum  Inputs=|-+
  Sum4 : Sum
  Sum5 : Sum  Inputs=|+-
  Switch : Switch  Threshold=1
  vehspdflow : Gain  Gain=0.01
  tag scope: AirFlowRequest=global, Heat_Reject_Eng=global
  wires:
  Data Type Conversion1/1 -> " "/1
  Cp of Air1/1 -> Q=Mc_air*Cp_air*delta T/3
  Switch/1 -> Q=Mc_air*Cp_air*delta T/2  "eng act air flow in kg/s"
  Q=Mc_air*Cp_air*delta T/1 -> " "/2  "J/s"
  " "/1 -> [Heat_Reject_Eng]  "J"
  Saturation/1 -> Sum3/1  "Actual air flow"
  Sum3/1 -> Compare To Zero/1
  Compare To Zero/1 -> Switch/2  "request meet"
  Cp of Air/1 -> "Eng Mc=Q/(Cp*delta T) "/2  "Cp J/kg*C"
  Ambient Temp/1 -> Sum5/2  "25 deg C"
  Sum5/1 -> Divide by Zero Fix/2(Divide), Q=Mc_air*Cp_air*delta T/1  "Delta T = Tcoolant - Tambient"
  EngCltTmp/1 -> Sum5/1  "EngCltTmp in deg C"
  "Eng Mc=Q/(Cp*delta T) "/1 -> Switch/1, Sum3/2, [AirFlowRequest]  "Eng requested air flow in Kg/s"
  Sum4/1 -> Switch/3, Saturation/1  "Air Flow Recieved"
  Fans/1 -> Data Type Conversion1/1
  [VehSpdAvgDrvn_Eng] -> vehspdflow/1
  vehspdflow/1 -> Sum4/2
  [Heat_Transfer_Eng] -> Divide by Zero Fix/1(Multiply)  "heat generation in w"
  Divide by Zero Fix/1(Output) -> "Eng Mc=Q/(Cp*delta T) "/1
  " "/1 -> Sum4/1
  Constant/1 -> " "/1

== system P2_SIL_Model_Diag/Camaro Plant Model/ICE Simple1/Inputs/Analog ==
  Constant : Constant
  Out1 : Outport
  wires:
  Constant/1 -> Out1/1

== system P2_SIL_Model_Diag/Camaro Plant Model/ICE Simple1/Inputs/CAN_from_HCU ==
  Bus Creator : BusCreator  Inputs=2
  Out1 : Outport
  wires:
  [HCU_to_EBCAN] -> Bus Creator/1
  [HCU_to_VEH_CAN] -> Bus Creator/2
  Bus Creator/1 -> Out1/1

== system P2_SIL_Model_Diag/Camaro Plant Model/ICE Simple1/Soft ECM/ECM_RollingAliveCnt ==
  Constant : Constant
  Rolling Alive Counter : Stateflow chart  TreatAsAtomicUnit=on
  Switch : Switch  Criteria=u2 > Threshold
  Out1 : Outport
  wires:
  [ECM_CAN_fault] -> Switch/2
  Constant/1 -> Switch/1
  Rolling Alive Counter/1(RollingAliveCnt) -> Switch/3
  Switch/1 -> Out1/1  "ECM_RollingAliveCnt"

== system P2_SIL_Model_Diag/Camaro Plant Model/ICE Simple1/Soft ECM/Fuel Consumption ==
  note: Total Fuel Consumed
  Fuel Consumption : Inport
  " " : Constant  Value=3600
  " tloop" : Constant  Value=0.01
  1/fuel density : Gain  Gain=1/(Engine.Fuel.Density*1000)
  Add : Sum  Inputs=|++
  Add1 : Sum  Inputs=|++
  Constant3 : Constant  Value=Engine.Fuel.Lower_Heating_Value/1000
  Divide : Product  Inputs=*/
  Divide by Zero Fix : Subsystem
  Divide by Zero Fix1 : Subsystem
  Memory : Memory
  Memory1 : Memory
  Product : Product  RndMeth=Zero
  Product1 : Product  RndMeth=Zero
  Product3 : Product  RndMeth=Zero
  Scope : Scope
  To Workspace5 : ToWorkspace  Commented=on  VariableName=eng_wh_per_mile_hist  SampleTime=-1
      settings: Decimation=WORKSPACE_DECIMATION
  fuel consumption : Outport
  wires:
  Divide by Zero Fix1/1(Output) -> To Workspace5/1
  Divide/1 -> Add1/1  "Wh"
  Memory1/1 -> Add1/2
  Add1/1 -> Divide by Zero Fix1/2(Multiply), Memory1/1  "cumulative"
  Product/1 -> Product3/2  "W"
  Constant3/1 -> Product/2
  Divide by Zero Fix/1(Output) -> fuel consumption/1, Scope/1
  [veh_dist_miles] -> Divide by Zero Fix1/1(Divide), Divide by Zero Fix/2(Multiply)  "miles"
  Product1/1 -> Add/1  "liter"
  1/fuel density/1 -> Product1/1  "liter/sec"
  Fuel Consumption/1 -> Product/1, 1/fuel density/1  "g/s"
  Memory/1 -> Add/2
  Add/1 -> Divide by Zero Fix/1(Divide), Memory/1  "cumulative_liter"
  " tloop"/1 -> Product3/1, Product1/2
  Product3/1 -> Divide/1
  " "/1 -> Divide/2

== system P2_SIL_Model_Diag/Camaro Plant Model/ICE Simple1/Soft ECM/Logic/APP2TP ==
  EngSpd : Inport
  APP : Inport  Port=2
  Shifter : Inport  Port=3
  f : TriggerPort  TriggerType=function-call  VariantControl=Variant
      settings: CopyFcn=Stateflow.SLINSF.SimulinkMan.removeBlockPreDeleteFcn  PreDeleteFcn=Stateflow.SLINSF.SimulinkMan.unsafePredeleteFcn
  Based on APP to TP test data from 2013 Malibu : Lookup_n-D  NumberOfTableDimensions=1  BreakpointsForDimension1=[0,1,2,3,4,5,6,7,8,9,10,11,12,13,14,15,16,17,18,19,20,21,22,23,24,25,26,27,28,29,30,31,32,33,34,35,36,37,38,39,40,41,42,43,44,45,46,48,51,55,60,66,100]  Table=[0,6.3,12.7686537241448,12.6326703204763,12.8888951657611,13.4307541011932,14.1739282202018,15.0532596030224,16.0198646102832,17.0384547356068,18.0848650172271,19.1437900086214,20.206727308158,21.2701286477589,22.3337585405773,23.3992604876916,24.4689307438132,25.5446996420107,26.6273204774486,27.7157659501418,28.8068321667249,29.8949502012373,30.9722052149229,32.0285631350456,33.0523048927199,34.0306682197568,34.9506970045247,35.8002982068255,36.5695063317874,37.2519554627699,37.846558853288,38.359396077948,38.8058077424007,39.2126977523099,39.6210431413345,40.0886114581279,40.6928857123509,41.5341968797017,42.7390639659588,44.4637416300428,46.8979753660875,50.2689642445339,54.8455312122302,60.9425009515619,68.9252852985734,79.2146762201353,81.9427,84.6943,87.2166,89.5096,91.3439,92.6051,100]  ExtrapMethod=Clip  UseLastTableValue=on  InternalRulePriority=Speed  RndMeth=Simplest  InputSameDT=on
  Compare To Constant1 : simulink/Logic and Bit Operations/Compare To Constant  relop=<  const=1  OutDataTypeStr=boolean
  Constant : Constant  Value=ParkGear
  Constant1 : Constant  Value=NeutralGear
  Constant2 : Constant  Value=Engine.IdleSpeed
  Display : Display
  "EngSpd " : InportShadow
  Kp : Gain  Gain=0.04
  Logical Operator : Logic  Operator=OR  AllPortsSameDT=off  OutDataTypeStr=boolean
  Logical Operator1 : Logic  AllPortsSameDT=off  OutDataTypeStr=boolean
  Product : Product
  RPM Derating : Lookup_n-D  NumberOfTableDimensions=1  BreakpointsForDimension1=[0 1000 2000 3000 4000 5000 6000 7000]  Table=[1 1 1 1 1 1 1 0]  ExtrapMethod=Clip  UseLastTableValue=on  InternalRulePriority=Speed  RndMeth=Simplest  InputSameDT=on
  Relational Operator : RelationalOperator  Operator===  OutDataTypeStr=boolean
  Relational Operator1 : RelationalOperator  Operator===  OutDataTypeStr=boolean
  Saturation : Saturate  UpperLimit=100  LowerLimit=0
  Sum : Sum  Inputs=|+-
  Switch : Switch  Threshold=1
  TP : Outport
  wires:
  Based on APP to TP test data from 2013 Malibu/1 -> Product/1  "1"
  Switch/1 -> TP/1
  EngSpd/1 -> RPM Derating/1
  RPM Derating/1 -> Product/2  "2"
  Shifter/1 -> Relational Operator/2, Relational Operator1/1
  Constant/1 -> Relational Operator/1
  Constant1/1 -> Relational Operator1/2
  Relational Operator/1 -> Logical Operator/1
  Relational Operator1/1 -> Logical Operator/2
  Logical Operator/1 -> Logical Operator1/1
  Constant2/1 -> Sum/1
  "EngSpd "/1 -> Sum/2
  Sum/1 -> Kp/1
  Kp/1 -> Saturation/1
  Saturation/1 -> Switch/1
  Logical Operator1/1 -> Switch/2  "Idle"
  Compare To Constant1/1 -> Logical Operator1/2
  APP/1 -> Display/1, Compare To Constant1/1, Based on APP to TP test data from 2013 Malibu/1  "3"
  Product/1 -> Switch/3

== system P2_SIL_Model_Diag/Camaro Plant Model/IMG/IMG Plant/ Actuators ==
  In1 : Inport
  Bus Selector : BusSelector  OutputSignals=MotTrqCmd,EngageClutch
  Out2 : Outport
  Out1 : Outport  Port=2
  wires:
  Bus Selector/1 -> Out2/1  "<MotTrqCmd>"
  In1/1 -> Bus Selector/1
  Bus Selector/2 -> Out1/1  "<EngageClutch>"

== system P2_SIL_Model_Diag/Camaro Plant Model/IMG/IMG Plant/Clutch ==
  clt_lockup_cmd : Inport
  clt_trq_in clt_inertia_in : Inport  Port=2
  clt_spd_out : Inport  Port=3
  Bus Creator : BusCreator  Inputs=2
  Bus Selector : BusSelector  OutputSignals=eng_trq_out_Nm,eng_inertia_out
  Inertia Calculaion : Subsystem
  Speed Calculaion : Subsystem
  Torque Calculaion : Subsystem
  clt_shaft_out : Outport
  ctl_spd_in : Outport  Port=2
  tag scope: clt_plant_spd_in=global, clt_plant_spd_out=global
  wires:
  clt_trq_in clt_inertia_in/1 -> Bus Selector/1
  Bus Creator/1 -> clt_shaft_out/1
  Inertia Calculaion/1(clutch out inertia) -> Bus Creator/2, [clt_plant_inertia_out]  "cpl_inertia_out"
  Torque Calculaion/1(clutch out trq) -> Bus Creator/1, [clt_plant_trq_out]  "clutch_trq_out"
  Speed Calculaion/1(clutch in spd) -> ctl_spd_in/1, [clt_plant_spd_in]
  clt_spd_out/1 -> [clt_plant_spd_out], Speed Calculaion/1(clutch out spd)
  Inertia Calculaion/2(clutch in inertia) -> Speed Calculaion/2(clutch in inertia)
  Bus Selector/1 -> [clt_plant_trq_in], Speed Calculaion/4(clutch in trq), Torque Calculaion/2(input trq)  "<eng_trq_out_Nm>"
  clt_lockup_cmd/1 -> [clt_plant_cmd], Speed Calculaion/3(lockup cmd), Inertia Calculaion/2(lockup cmd), Torque Calculaion/1(lockup cmd)
  Bus Selector/2 -> [clt_plant_inertia_in], Inertia Calculaion/1(inertia in)  "<eng_inertia_out>"

== system P2_SIL_Model_Diag/Camaro Plant Model/IMG/IMG Plant/Electric Machine ==
  MotTrqCmd : Inport
  voltage : Inport  Port=2
  mot_trq_in mot_inertia_in : Inport  Port=3
  MotSpdOut : Inport  Port=4
  Bus Creator : BusCreator  Inputs=2
  Bus Selector : BusSelector  OutputSignals=clutch_trq_out,cpl_inertia_out
  "Calculate Mot Efficiency, MotPwrMech, and, MotPwrElec" : Subsystem
  Constant : Constant  Value=0
  Gain : Gain  Gain=2
  Inertia (kg-m^2) : Constant  Value=mot.plant.init.inertia
  MotTrqExcessTrigger : Subsystem
  Sum : Sum  Inputs=|++
  Sum1 : Sum  Inputs=++|
  Sum2 : Sum  Inputs=|++
  Switch : Switch  Criteria=u2 > Threshold
  Switch1 : Switch  Threshold=1
  Thermal : Subsystem
  Torque Calculation : Subsystem
  non-zero division : Subsystem
      mask Display: disp('divider \n I1/I2')
  voltage1 : InportShadow  Port=2
  mot_current_out : Outport
  mot_trq_out mot_inertia_out : Outport  Port=2
  MotSpdIn : Outport  Port=3
  tag scope: mcu_temp=global, mot_crr_out=global, mot_spd_out=global, mot_temp=global, mot_trq_out=global, mot_volt_in=global
  wires:
  voltage/1 -> [mot_volt_in], non-zero division/2(In2)
  "Calculate Mot Efficiency, MotPwrMech, and, MotPwrElec"/2(MotPwrElec) -> non-zero division/1(In1)  "Pelec"
  non-zero division/1(Out1) -> [mot_crr_out], mot_current_out/1
  Bus Creator/1 -> mot_trq_out mot_inertia_out/1
  Sum/1 -> Bus Creator/2  "mot_inertia_out"
  mot_trq_in mot_inertia_in/1 -> Bus Selector/1
  Bus Selector/1 -> Sum1/2  "<clutch_trq_out>"
  Bus Selector/2 -> Sum/1  "<cpl_inertia_out>"
  Inertia (kg-m^2)/1 -> Sum/2
  Sum1/1 -> Bus Creator/1  "mot_trq_out"
  "Calculate Mot Efficiency, MotPwrMech, and, MotPwrElec"/1(Losses) -> Thermal/1(Losses)
  MotTrqCmd/1 -> Torque Calculation/2(MotTrqCmd)
  MotSpdOut/1 -> [mot_spd_out], "Calculate Mot Efficiency, MotPwrMech, and, MotPwrElec"/1(MotSpd), MotSpdIn/1, Torque Calculation/1(MotSpd)
  Thermal/1(mot_temp_C) -> Gain/1, Switch1/3
  voltage1/1 -> Switch/2
  Constant/1 -> Switch/3
  MotTrqExcessTrigger/1(Out1) -> Sum1/1, "Calculate Mot Efficiency, MotPwrMech, and, MotPwrElec"/2(MotTrqAct)
  "Calculate Mot Efficiency, MotPwrMech, and, MotPwrElec"/3(MCU_Temp) -> [mcu_temp]
  [MotOverTemp] -> Switch1/2
  Gain/1 -> Switch1/1
  Switch1/1 -> [mot_temp]
  Switch/1 -> MotTrqExcessTrigger/1(In1), [mot_trq_out]
  [MotTrqMismatch] -> Sum2/1
  Torque Calculation/1(mot_trq_out) -> Sum2/2
  Sum2/1 -> Switch/1

== system P2_SIL_Model_Diag/Camaro Plant Model/IMG/IMG Plant/Sensors ==
  In2 : Inport
  In3 : Inport  Port=2
  In4 : Inport  Port=3
  In5 : Inport  Port=4
  In6 : Inport  Port=5
  In1 : Inport  Port=6
  In7 : Inport  Port=7
  Bus Creator : BusCreator  Inputs=7
  Out1 : Outport
  wires:
  In6/1 -> Bus Creator/5  "mot_temp"
  In3/1 -> Bus Creator/2  "mot_trq_out"
  In5/1 -> Bus Creator/4  "mot_volt_in"
  In4/1 -> Bus Creator/3  "mot_crr_out"
  In2/1 -> Bus Creator/1  "mot_spd_out"
  Bus Creator/1 -> Out1/1
  In1/1 -> Bus Creator/6  "mcu_temp"
  In7/1 -> Bus Creator/7  "clt_plant_spd_in"

== system P2_SIL_Model_Diag/Camaro Plant Model/IMG/Soft MCU/MCU_CAN_rolling ==
  Constant8 : Constant
  Rolling Alive Counter1 : Stateflow chart  TreatAsAtomicUnit=on
  Switch1 : Switch  Criteria=u2 > Threshold
  Out1 : Outport
  wires:
  Switch1/1 -> Out1/1  "MCURollingAliveCnt [0 1 2 3]"
  [MCU_CAN_fault] -> Switch1/2
  Constant8/1 -> Switch1/1
  Rolling Alive Counter1/1(RollingAliveCnt) -> Switch1/3

== system P2_SIL_Model_Diag/Camaro Plant Model/IMG/Soft MCU/Torque Calculation ==
  MotTrqReq : Inport
  MotSpd : Inport  Port=2
  MotTrqFdbck : Inport  Port=3
  Abs : Abs
  Abs1 : Abs
  MinMax : MinMax  Inputs=2
  Product : Product
  Sign : Signum
  "max torque " : Subsystem
  mot_trq_out : Outport
  wires:
  Product/1 -> mot_trq_out/1
  "max torque "/1(max torque) -> Abs1/1
  MotSpd/1 -> "max torque "/2(speed)
  MotTrqReq/1 -> "max torque "/1(Req), Sign/1, Abs/1
  Sign/1 -> Product/1
  MinMax/1 -> Product/2
  Abs/1 -> MinMax/1
  Abs1/1 -> MinMax/2
  MotTrqFdbck/1 -> "max torque "/3(torque)

== system P2_SIL_Model_Diag/Camaro Plant Model/On-Board Charger/HCU to OBC/CAN_fromHCU ==
  Outputs : Outport
  wires:
  [HCU_to_HV_CAN] -> Outputs/1

== system P2_SIL_Model_Diag/Camaro Plant Model/On-Board Charger/HCU to OBC/Digital_fromHCU ==
  Outputs : Outport
  wires:
  [Digital] -> Outputs/1

== system P2_SIL_Model_Diag/Camaro Plant Model/On-Board Charger/On Board Charger/ Actuators ==
  In1 : Inport
  Bus Selector : BusSelector  OutputSignals=Enable,NLG5_MC_MAX,NLG5_OC_COM,VoltageEnable
  Out2 : Outport
  Out1 : Outport  Port=2
  Out3 : Outport  Port=3
  Out4 : Outport  Port=4
  wires:
  Bus Selector/1 -> Out2/1  "<Enable>"
  In1/1 -> Bus Selector/1
  Bus Selector/2 -> Out1/1  "<NLG5_MC_MAX>"
  Bus Selector/3 -> Out3/1  "<NLG5_OC_COM>"
  Bus Selector/4 -> Out4/1  "<VoltageEnable>"

== system P2_SIL_Model_Diag/Camaro Plant Model/On-Board Charger/On Board Charger/Sensors ==
  In2 : Inport
  In3 : Inport  Port=2
  In4 : Inport  Port=3
  In5 : Inport  Port=4
  Bus Creator : BusCreator  Inputs=4
  Out1 : Outport
  wires:
  In3/1 -> Bus Creator/2  "ActOutCrnt"
  In5/1 -> Bus Creator/4  "OBCTemp"
  In4/1 -> Bus Creator/3  "MainsVoltage"
  In2/1 -> Bus Creator/1  "BatteryVoltage"
  Bus Creator/1 -> Out1/1

== system P2_SIL_Model_Diag/Camaro Plant Model/On-Board Charger/On Board Charger/Subsystem2 ==
  In1 : Inport
  In2 : Inport  Port=2
  Fcn : Fcn  Expr=u[1]/(u[2]+eps)*(u[2]!=0)
  Mux : Mux  Inputs=2
  Out1 : Outport
  wires:
  In2/1 -> Mux/2
  Fcn/1 -> Out1/1
  In1/1 -> Mux/1
  Mux/1 -> Fcn/1

== system P2_SIL_Model_Diag/Camaro Plant Model/On-Board Charger/Soft_OBC/NLG5_ACT_I ==
  Bus Creator : BusCreator  Inputs=4
  Divide_by_Zero_Fix : EC2_libraries/Divide_by_Zero_Fix  Commented=on
  Efficiency : Constant  Commented=on  Value=obc.plant.init.avergae_efficiency
  From5 : From  Commented=on  GotoTag=NLG5_MV_ACT  TagVisibility=global
  From6 : From  Commented=on  GotoTag=NLG5_OC_ACT  TagVisibility=global
  From7 : From  Commented=on  GotoTag=NLG5_OV_ACT  TagVisibility=global
  NLG5_MC_ACT : Constant
  V*I : Product  Commented=on  Inputs=**/  RndMeth=Zero
  NLG5_ACT_I : Outport
  wires:
  From5/1 -> Divide_by_Zero_Fix/2
  V*I/1 -> Divide_by_Zero_Fix/1
  Efficiency/1 -> V*I/3
  [NLG5_OV_ACT] -> Bus Creator/3  "NLG5_OV_ACT"
  [NLG5_OC_ACT] -> Bus Creator/4  "NLG5_OC_ACT"
  [NLG5_MV_ACT] -> Bus Creator/2  "NLG5_MV_ACT"
  Bus Creator/1 -> NLG5_ACT_I/1  "NLG5_ACT_I"
  From6/1 -> V*I/2
  From7/1 -> V*I/1
  NLG5_MC_ACT/1 -> Bus Creator/1

== system P2_SIL_Model_Diag/Camaro Plant Model/On-Board Charger/Soft_OBC/NLG5_ACT_II ==
  Bus Creator : BusCreator  Inputs=5
  Constant{1..4} (4 alike) : Constant  Value=0
  Constant6 : Constant  Value=obc.plant.init.Maximum_Mains_Current
  NLG5_ACT_II : Outport
  wires:
  Constant4/1 -> Bus Creator/5  "NLG5_OC_BO"
  Bus Creator/1 -> NLG5_ACT_II/1  "NLG5_ACT_II"
  Constant6/1 -> Bus Creator/1  "NLG5_S_MC_M_CP"
  Constant1/1 -> Bus Creator/2  "NLG5_S_MC_M_PI"
  Constant3/1 -> Bus Creator/4  "NLG5_AHC_EXT"
  Constant2/1 -> Bus Creator/3  "NLG5_ABV"
